simulink model "P_SP_paramEst"  (R2020a)
settings: Solver=FixedStepAuto  StartTime=0.0  StopTime=100  FixedStep=0.01  RelTol=1e-3
InitFcn:
  | variableLoad
values from neighbouring files (symbols this model uses):
  a = 1    [variableLoad.m]
  a_m = 0.8    [variableLoad.m]
  b = 2    [variableLoad.m]
  eMax = 0.3    [variableLoad.m]
libraries: cstblocks x2, simulink x1
settings Model: Creator=alfystar  LastModifiedBy=alfystar

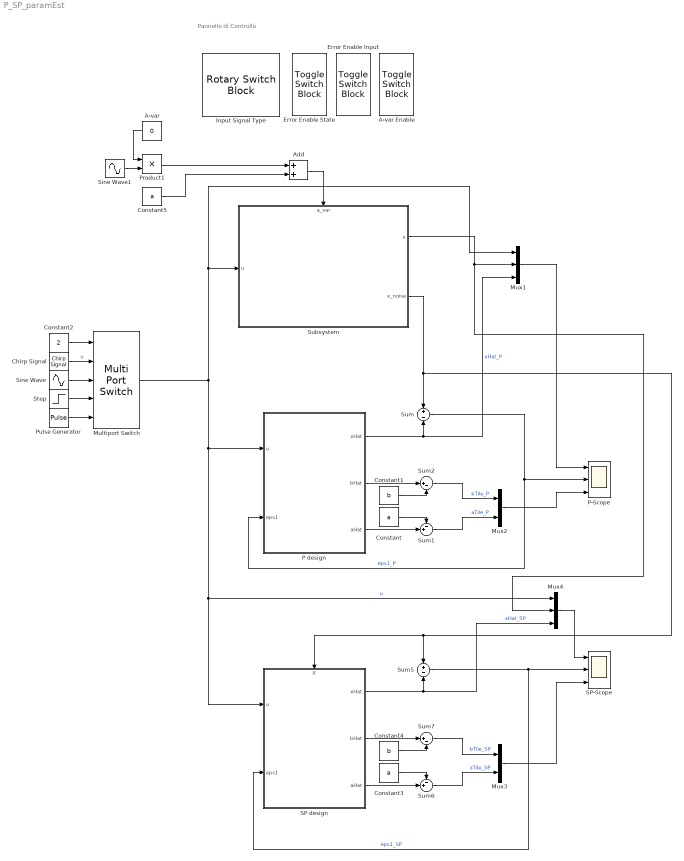
== system P_SP_paramEst ==
  note: Pannello di Controllo
  A-var : Constant  Value=0
  A-var Enable : ToggleSwitchBlock
      settings: Values={{'Error-Off', 'Error-On'}, [0 1]}
  Add : Sum
  Chirp Signal : simulink/Sources/Chirp Signal  f1=0.1  T=100  f2=1
  Constant : Constant  Value=a
  Constant1 : Constant  Value=b
  Constant2 : Constant  Value=2
  Constant3 : Constant  Value=a
  Constant4 : Constant  Value=b
  Constant5 : Constant  Value=a
  Error Enable Input : ToggleSwitchBlock
      settings: Values={{'Error-Off', 'Error-On'}, [0 1]}
  Error Enable State : ToggleSwitchBlock
      settings: Values={{'Error-Off', 'Error-On'}, [0 1]}
  Input Signal Type : RotarySwitchBlock
      settings: Values={{'Chirp', 'Sine', 'Step', 'Impulse'}, [1 2 3 4]}
  Multiport Switch : MultiPortSwitch  DataPortOrder=Specify indices  DataPortIndices={1,2,3,4}
  Mux1 : Mux  Inputs=3
  Mux2 : Mux  Inputs=2
  Mux3 : Mux  Inputs=2
  Mux4 : Mux  Inputs=3
  P design : Subsystem
  P-Scope : Scope  NumInputPorts=3
  Product1 : Product
  Pulse Generator : DiscretePulseGenerator  PulseType=Time based  Amplitude=10  PulseWidth=5
  SP design : Subsystem
      settings: PortSchema="{\"entries\":[{\"content\":{\"sides\":[{\"content\":{\"connectorIds\":[\"In1\",\"In2\"]},\"type\":\"ConnectorPlacement.EquallySpacedRectSide\",\"uuid\":\"e9709b4b-489e-426b-86db-a8a5b46a3381\"},{\"content\":{\"connectorIds\":[\"Out1\",\"Out2\",\"Out3\"],\"side\":\"RIGHT\"},\"type\":\"ConnectorPlacement.EquallySpacedRectSide\",\"uuid\":\"298f9992-e7ab-4ae3-9bf7-5a2add14c94f\"},{\"content\":{\"connectorIds\":[\"In3\"],\"side\":\"TOP\"},\"type\":\"ConnectorPlacement.EquallySpacedRectSide\",\"uuid\":\"de1e1138-6363-4f2b-8530-3bd0c6039d48\"},{\"content\":{\"connectorIds\":[],\"side\":\"BOTTOM\"},\"type\":\"ConnectorPlacement.EquallySpacedRectSide\",\"uuid\":\"e8a343d9-6c18-4903-865a-d456b3dfa344\"}]},\"type\":\"ConnectorPlacement.EquallySpacedConnector\",\"uuid\":\"a8e0b7e6-aa41-477f-a5f6-9bff79cc4341\"}],\"packageUris\":[\"http://schema.mathworks.com/mf0/Connector/19700101\"],\"version\":\"1.0\"}"
  SP-Scope : Scope  NumInputPorts=3
  Sine Wave : Sin  SampleTime=0
  Sine Wave1 : Sin  Amplitude=0.1  Frequency=2*pi/(24*3600)  SampleTime=0
  Step : Step  SampleTime=0
  Subsystem : Subsystem
      settings: PortSchema="{\"entries\":[{\"content\":{\"sides\":[{\"content\":{\"connectorIds\":[\"In1\"]},\"type\":\"ConnectorPlacement.EquallySpacedRectSide\",\"uuid\":\"14635710-82f9-4a65-bcc0-83f1e09f878c\"},{\"content\":{\"connectorIds\":[\"Out1\",\"Out2\"],\"side\":\"RIGHT\"},\"type\":\"ConnectorPlacement.EquallySpacedRectSide\",\"uuid\":\"452a6707-d8f6-41ed-98e8-a047019bdffe\"},{\"content\":{\"connectorIds\":[\"In2\"],\"side\":\"TOP\"},\"type\":\"ConnectorPlacement.EquallySpacedRectSide\",\"uuid\":\"b27a105c-a632-4888-a681-744510874af5\"}]},\"type\":\"ConnectorPlacement.EquallySpacedConnector\",\"uuid\":\"15183480-a8b0-4184-a294-65d7280436a8\"}],\"packageUris\":[\"http://schema.mathworks.com/mf0/Connector/19700101\"],\"version\":\"1.0\"}"
  Sum : Sum  Inputs=+|-
  Sum1 : Sum  Inputs=-+|
  Sum2 : Sum  Inputs=|+-
  Sum5 : Sum  Inputs=+|-
  Sum6 : Sum  Inputs=-+|
  Sum7 : Sum  Inputs=|+-
  wires:
  Sum/1 -> P design/2(eps1), P-Scope/2  "eps1_P"
  P design/1(xHat) -> Mux1/3, Sum/2  "xHat_P"
  Mux1/1 -> P-Scope/1
  Constant/1 -> Sum1/1
  P design/3(aHat) -> Sum1/2
  Sum1/1 -> Mux2/2  "aTile_P"
  Constant1/1 -> Sum2/2
  P design/2(bHat) -> Sum2/1
  Sum2/1 -> Mux2/1  "bTile_P"
  Mux2/1 -> P-Scope/3
  Step/1 -> Multiport Switch/4
  Constant2/1 -> Multiport Switch/1
  Pulse Generator/1 -> Multiport Switch/5
  Sine Wave/1 -> Multiport Switch/3
  Chirp Signal/1 -> Multiport Switch/2  "u"
  SP design/3(aHat) -> Sum6/2
  Mux3/1 -> SP-Scope/3
  SP design/2(bHat) -> Sum7/1
  Sum7/1 -> Mux3/1  "bTile_SP"
  Sum6/1 -> Mux3/2  "aTile_SP"
  Multiport Switch/1 -> Mux4/1, SP design/1(u), P design/1(u), Mux1/1, Subsystem/1(u)  "u"
  Sum5/1 -> SP design/2(eps1), SP-Scope/2  "eps1_SP"
  SP design/1(xHat) -> Mux4/3, Sum5/2  "xHat_SP"
  Constant3/1 -> Sum6/1
  Constant4/1 -> Sum7/2
  Mux4/1 -> SP-Scope/1
  Subsystem/1(x) -> Mux4/2, Mux1/2
  Subsystem/2(x_noise) -> SP design/3(X), Sum5/1, Sum/1
  A-var/1 -> Product1/1
  Sine Wave1/1 -> Product1/2
  Add/1 -> Subsystem/2(a_var)
  Product1/1 -> Add/1
  Constant5/1 -> Add/2

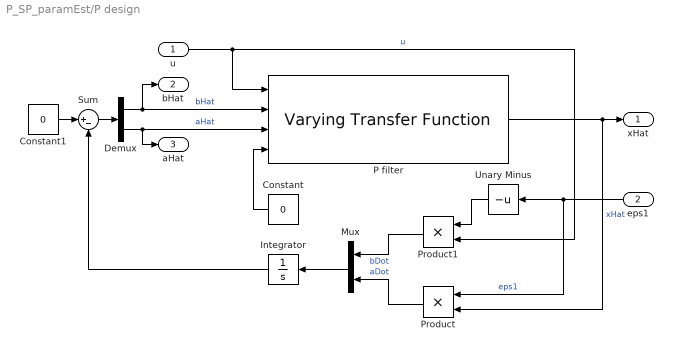
== system P_SP_paramEst/P design ==
  u : Inport
  eps1 : Inport  Port=2
  Constant : Constant  Value=0
  Constant1 : Constant  Value=0
  Demux : Demux  Outputs=2
  Integrator : Integrator
  Mux : Mux  Inputs=2
  P filter : cstblocks/Linear Parameter Varying/Varying Transfer Function  N=1
  Product : Product
  Product1 : Product
  Sum : Sum  Inputs=|+-
  Unary Minus : UnaryMinus
  xHat : Outport
  bHat : Outport  Port=2
  aHat : Outport  Port=3
  wires:
  u/1 -> P filter/1, Product1/2  "u"
  eps1/1 -> Product/1, Unary Minus/1  "eps1"
  P filter/1 -> Product/2, xHat/1  "xHat"
  Constant/1 -> P filter/4
  Mux/1 -> Integrator/1
  Sum/1 -> Demux/1
  Constant1/1 -> Sum/1
  Integrator/1 -> Sum/2
  Demux/1 -> bHat/1, P filter/2  "bHat"
  Demux/2 -> aHat/1, P filter/3  "aHat"
  Unary Minus/1 -> Product1/1
  Product1/1 -> Mux/1  "bDot"
  Product/1 -> Mux/2  "aDot"

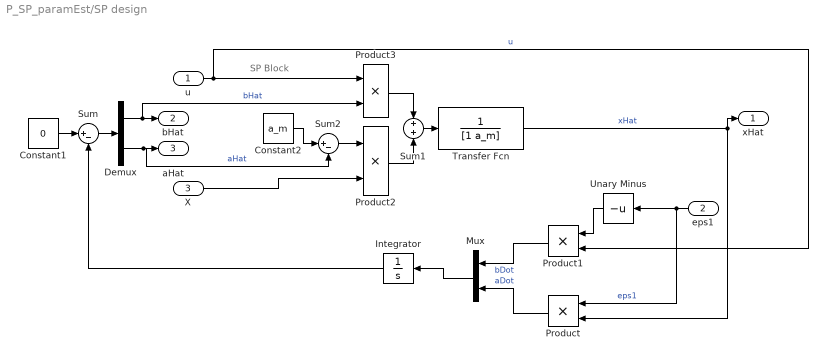
== system P_SP_paramEst/SP design ==
  note: SP Block
  u : Inport
  eps1 : Inport  Port=2
  X : Inport  Port=3
  Constant1 : Constant  Value=0
  Constant2 : Constant  Value=a_m
  Demux : Demux  Outputs=2
  Integrator : Integrator
  Mux : Mux  Inputs=2
  Product{,1..3} (4 alike) : Product
  Sum : Sum  Inputs=|+-
  Sum1 : Sum  Inputs=+|+
  Sum2 : Sum  Inputs=|+-
  Transfer Fcn : TransferFcn  Denominator=[1 a_m]
  Unary Minus : UnaryMinus
  xHat : Outport
  bHat : Outport  Port=2
  aHat : Outport  Port=3
  wires:
  u/1 -> Product1/2, Product3/1  "u"
  eps1/1 -> Product/1, Unary Minus/1  "eps1"
  Transfer Fcn/1 -> Product/2, xHat/1  "xHat"
  Mux/1 -> Integrator/1
  Sum/1 -> Demux/1
  Constant1/1 -> Sum/1
  Integrator/1 -> Sum/2
  Demux/1 -> Product3/2, bHat/1  "bHat"
  Demux/2 -> Sum2/2, aHat/1  "aHat"
  Unary Minus/1 -> Product1/1
  Product1/1 -> Mux/1  "bDot"
  Product/1 -> Mux/2  "aDot"
  Sum1/1 -> Transfer Fcn/1
  X/1 -> Product2/2
  Product2/1 -> Sum1/2
  Constant2/1 -> Sum2/1
  Sum2/1 -> Product2/1
  Product3/1 -> Sum1/1

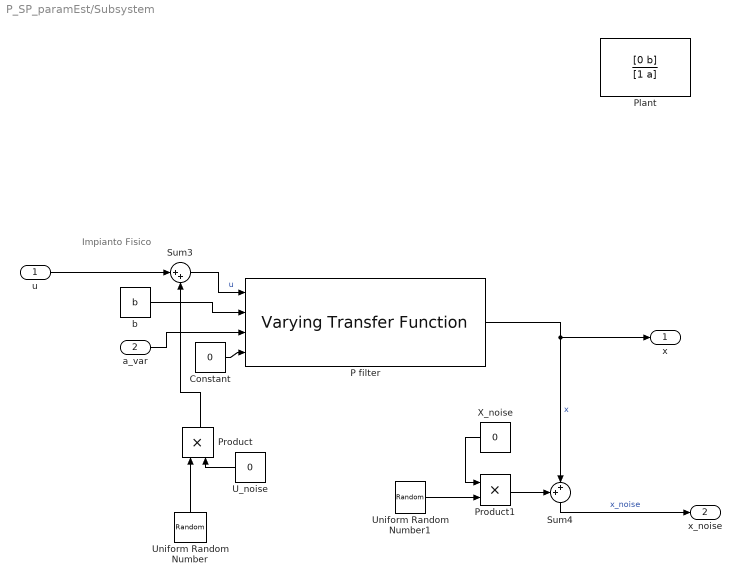
== system P_SP_paramEst/Subsystem ==
  note: Impianto Fisico
  u : Inport
  a_var : Inport  Port=2
  Constant : Constant  Value=0
  P filter : cstblocks/Linear Parameter Varying/Varying Transfer Function  N=1
  Plant : TransferFcn  Numerator=[0 b]  Denominator=[1 a]
  Product : Product
  Product1 : Product
  Sum3 : Sum  Inputs=|++
  Sum4 : Sum  Inputs=++|
  U_noise : Constant  Value=0
  Uniform Random Number : UniformRandomNumber  Minimum=-eMax  Maximum=eMax  SampleTime=0.1
  Uniform Random Number1 : UniformRandomNumber  Minimum=-eMax  Maximum=eMax  SampleTime=0.1
  X_noise : Constant  Value=0
  b : Constant  Value=b
  x : Outport
  x_noise : Outport  Port=2
  wires:
  Uniform Random Number1/1 -> Product1/2
  P filter/1 -> Sum4/2, x/1  "x"
  Product/1 -> Sum3/2
  X_noise/1 -> Product1/1
  Sum4/1 -> x_noise/1  "x_noise"
  Sum3/1 -> P filter/1  "u"
  Uniform Random Number/1 -> Product/1
  u/1 -> Sum3/1
  Product1/1 -> Sum4/1
  U_noise/1 -> Product/2
  a_var/1 -> P filter/3
  Constant/1 -> P filter/4
  b/1 -> P filter/2
